simulink model "LinearTimeInvariant_CHECKED"  (Simulink 8.0)
settings: Solver=ode45  StartTime=0.0  StopTime=10.0  RelTol=1e-3
undefined symbols (not defined in the file or in its folder): Aii, Aij, Bi
settings Model: Creator=chepeadan  LastModifiedBy=trommsdorff
settings DataIOCC: SignalLoggingSaveFormat=ModelDataLogs
settings DebuggingCC: FcnCallInpInsideContextMsg=UseLocalSettings  StrictBusMsg=Warning
settings GRTTargetCC: CombineOutputUpdateFcns=off  GRTInterface=on

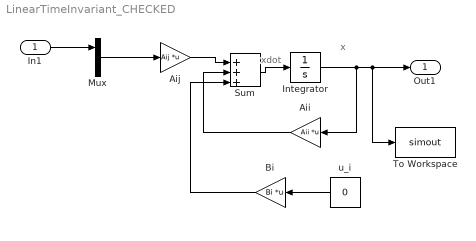
== system LinearTimeInvariant_CHECKED ==
  note: xdot
  note: x
  In1 : Inport
  Aii : Gain  Gain=Aii  Multiplication=Matrix(K*u) (u vector)
  Aij : Gain  Gain=Aij  Multiplication=Matrix(K*u) (u vector)
  Bi : Gain  Gain=Bi  Multiplication=Matrix(K*u) (u vector)
  Integrator : Integrator
  Mux : Mux  Inputs=2
  Sum : Sum  Inputs=|+|+|+
  To Workspace : ToWorkspace  VariableName=simout  SampleTime=-1  SaveFormat=Structure With Time
  u_i : Constant  Value=0
  Out1 : Outport
  wires:
  In1/1 -> Mux/1
  Integrator/1 -> Aii/1, Out1/1, To Workspace/1
  Mux/1 -> Aij/1
  Aij/1 -> Sum/1
  Aii/1 -> Sum/2
  u_i/1 -> Bi/1
  Bi/1 -> Sum/3
  Sum/1 -> Integrator/1
